simulink model "Pleural_Schuessler"  (Simulink 6.4)
settings: Solver=ode45  StartTime=0.0  StopTime=10.0  RelTol=1e-3
values from neighbouring files (symbols this model uses):
  E_CW = 5    [Pleural_Schuessler_IC.m]    (also in Pmus_Flow_Younes_IC.m; Resp_Mech_IC.m; Respiratory_IC.m)
  kaw1 = 1.85    [Pleural_Schuessler_IC.m]    (also in Resp_Mech_IC.m; Respiratory_IC.m)
  kaw2 = 0.43    [Pleural_Schuessler_IC.m]    (also in Resp_Mech_IC.m; Respiratory_IC.m)
  R_CW = 1.03    [Pleural_Schuessler_IC.m]    (also in Pmus_Flow_Younes_IC.m; Resp_Mech_IC.m; Respiratory_IC.m)
settings Model: LastModifiedBy=CLM
settings OptimizationCC: BlockReduction=off  BooleanDataType=off
settings DebuggingCC: SolverPrmCheckMsg=none  StrictBusMsg=None
settings HardwareCC: TargetUnknown=on

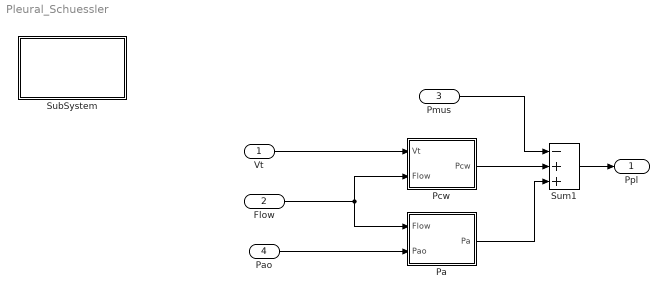
== system Pleural_Schuessler ==
  Vt : Inport
  Flow : Inport  Port=2
  "Pmus " : Inport  Port=3
  "Pao " : Inport  Port=4
  Pa : Subsystem
  Pcw : Subsystem
  SubSystem : Subsystem
      settings: OpenFcn=Pleural_Schuessler_IC
      mask Display: disp('"double click here"\n to load \nPleural_Schuessler \ninitial values');
  Sum1 : Sum  Inputs=-++  SaturateOnIntegerOverflow=on  InputSameDT=on
  "Ppl " : Outport
  wires:
  Sum1/1 -> "Ppl "/1
  Flow/1 -> Pa/1("Flow   "), Pcw/2(Flow)
  "Pao "/1 -> Pa/2("Pao ")
  Vt/1 -> Pcw/1(Vt)
  Pcw/1("Pcw  ") -> Sum1/2
  "Pmus "/1 -> Sum1/1
  Pa/1("Pa ") -> Sum1/3

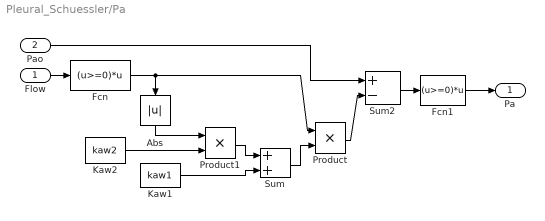
== system Pleural_Schuessler/Pa ==
  "Flow   " : Inport
  "Pao " : Inport  Port=2
  Abs : Abs  Orientation=down  SaturateOnIntegerOverflow=on  SampleTime=-1
  Fcn : Fcn  Expr=(u>=0)*u
  Fcn1 : Fcn  Expr=(u>=0)*u
  "Kaw1 " : Constant  Value=kaw1  OutDataType=sfix(16)  ConRadixGroup=Use specified scaling  OutScaling=2^0  SampleTime=inf  FramePeriod=inf
  "Kaw2 " : Constant  Value=kaw2  OutDataType=sfix(16)  ConRadixGroup=Use specified scaling  OutScaling=2^0  SampleTime=inf  FramePeriod=inf
  Product : Product  SaturateOnIntegerOverflow=on  RndMeth=Zero  InputSameDT=on
  Product1 : Product  SaturateOnIntegerOverflow=on  RndMeth=Zero  InputSameDT=on
  Sum : Sum  SaturateOnIntegerOverflow=on  InputSameDT=on
  Sum2 : Sum  Inputs=+-  SaturateOnIntegerOverflow=on  InputSameDT=on
  "Pa " : Outport
  wires:
  Fcn1/1 -> "Pa "/1
  Product/1 -> Sum2/2
  Sum2/1 -> Fcn1/1
  "Pao "/1 -> Sum2/1
  Fcn/1 -> Product/1, Abs/1
  "Flow   "/1 -> Fcn/1
  Sum/1 -> Product/2
  "Kaw1 "/1 -> Sum/2
  Product1/1 -> Sum/1
  Abs/1 -> Product1/1
  "Kaw2 "/1 -> Product1/2

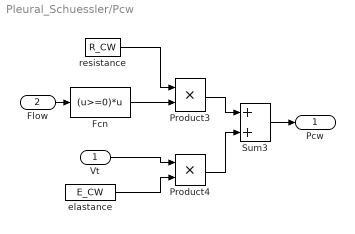
== system Pleural_Schuessler/Pcw ==
  Vt : Inport
  Flow : Inport  Port=2
  Fcn : Fcn  Expr=(u>=0)*u
  Product3 : Product  SaturateOnIntegerOverflow=on  RndMeth=Zero  InputSameDT=on
  Product4 : Product  SaturateOnIntegerOverflow=on  RndMeth=Zero  InputSameDT=on
  Sum3 : Sum  SaturateOnIntegerOverflow=on  InputSameDT=on
  elastance : Constant  Value=E_CW  OutDataType=sfix(16)  ConRadixGroup=Use specified scaling  OutScaling=2^0  SampleTime=inf  FramePeriod=inf
  "resistance " : Constant  Value=R_CW  OutDataType=sfix(16)  ConRadixGroup=Use specified scaling  OutScaling=2^0  SampleTime=inf  FramePeriod=inf
  "Pcw  " : Outport
  wires:
  "resistance "/1 -> Product3/1
  Product3/1 -> Sum3/1
  Flow/1 -> Fcn/1
  Product4/1 -> Sum3/2
  Sum3/1 -> "Pcw  "/1
  elastance/1 -> Product4/2
  Vt/1 -> Product4/1
  Fcn/1 -> Product3/2

== system Pleural_Schuessler/SubSystem ==
